simulink model "L4"  (R2016b)
settings: Solver=FixedStepAuto  StartTime=0.0  StopTime=20  FixedStep=0.05  RelTol=1e-3
values from neighbouring files (symbols this model uses):
  global_path_heading = zeros(1,num1)    [referenceline.m]
  global_path_kappa = zeros(1,num1)    [referenceline.m]
  global_path_x = 0: 0.2 : LaneLength    [Map.m]    (also in referenceline.m)
  global_path_y = zeros(1,num1)    [Map.m]    (also in referenceline.m)
(part 1 of 4)
settings Model: Creator=Administrator  LastModifiedBy=Administrator

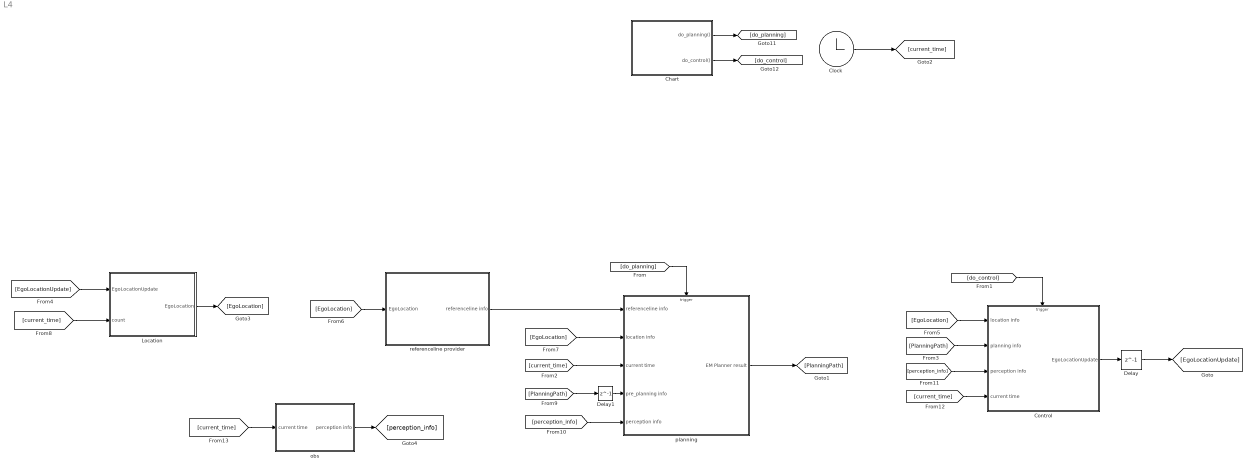
== system L4 ==
  Chart : Stateflow chart  TreatAsAtomicUnit=on
  Clock : Clock
  Control : Subsystem  TreatAsAtomicUnit=on
  Delay : Delay  DelayLength=1  InitialCondition=0
  Delay1 : Delay  DelayLength=1  InitialCondition=0
  Location : Subsystem
  obs : Subsystem
  planning : Subsystem  TreatAsAtomicUnit=on
  referenceline provider : Subsystem
  wires:
  Chart/2(do_control()) -> [do_control]
  Chart/1(do_planning()) -> [do_planning]
  [do_planning] -> planning/Trigger
  [do_control] -> Control/Trigger
  Clock/1 -> [current_time]
  [current_time] -> Location/2(count)
  Control/1(EgoLocationUpdate) -> Delay/1
  [EgoLocationUpdate] -> Location/1(EgoLocationUpdate)
  [PlanningPath] -> Control/2(planning info)
  Location/1(EgoLocation) -> [EgoLocation]
  [EgoLocation] -> Control/1(location info)
  [EgoLocation] -> referenceline provider/1(EgoLocation)
  [EgoLocation] -> planning/2(location info)
  [current_time] -> planning/3(current time)
  referenceline provider/1(referenceline info) -> planning/1(referenceline info)
  planning/1(EM Planner result) -> [PlanningPath]
  [PlanningPath] -> Delay1/1
  Delay1/1 -> planning/4(pre_planning info)
  obs/1(perception info) -> [perception_info]
  [perception_info] -> planning/5(perception info)
  [perception_info] -> Control/3(perception info)
  [current_time] -> Control/4(current time)
  Delay/1 -> [EgoLocationUpdate]
  [current_time] -> obs/1(current time)

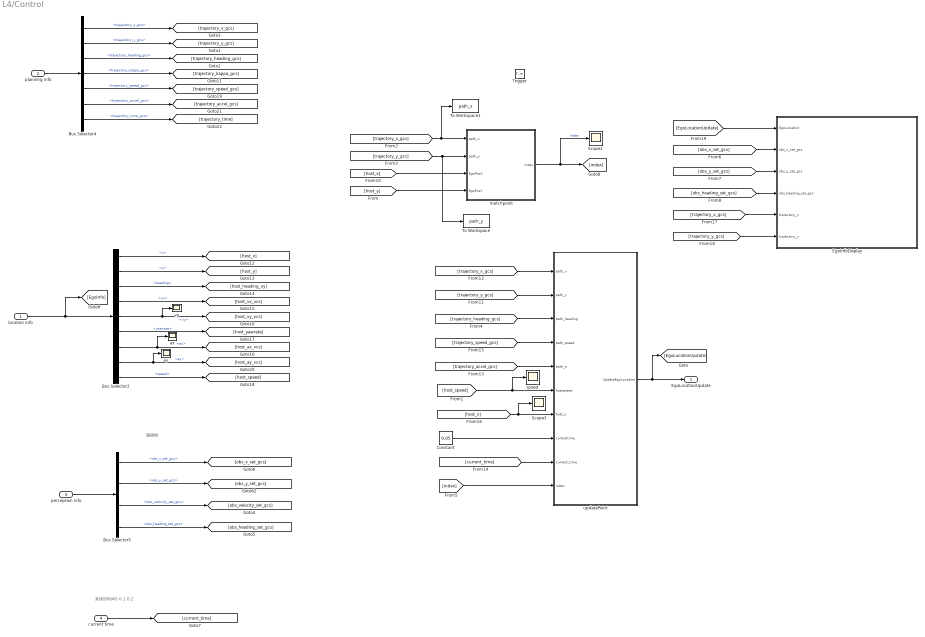
== system L4/Control ==
  note: 障碍物
  note: 系统的时间0 0.1 0.2
  location info : Inport
  planning info : Inport  Port=2
  perception info : Inport  Port=3
  current time : Inport  Port=4
  Trigger : TriggerPort  TriggerType=function-call  VariantControl=Variant
  Bus Selector2 : BusSelector  OutputSignals=x,y,heading,vx,vy,yawrate,ax,ay,speed
  Bus Selector4 : BusSelector  OutputSignals=trajectory_x_gcs,trajectory_y_gcs,trajectory_heading_gcs,trajectory_kappa_gcs,trajectory_speed_gcs,trajectory_accel_gcs,trajectory_time_gcs
  Bus Selector5 : BusSelector  OutputSignals=obs_x_set_gcs,obs_y_set_gcs,obs_velocity_set_gcs,obs_heading_set_gcs
  Constant : Constant  Value=0.05
  EgoInfoDisplay : MATLAB Function  TreatAsAtomicUnit=on
  Scope1 : Scope
  Scope3 : Scope
  To Workspace : ToWorkspace  VariableName=path_y  SampleTime=-1
  To Workspace1 : ToWorkspace  VariableName=path_x  SampleTime=-1
  ax : Scope
  ay : Scope
  matchpoint : MATLAB Function  TreatAsAtomicUnit=on
  speed : Scope
  updatePoint : MATLAB Function  TreatAsAtomicUnit=on
  vy : Scope
  EgoLocationUpdate : Outport
  wires:
  [host_x] -> matchpoint/3(EgoPosX)
  [host_y] -> matchpoint/4(EgoPosY)
  [trajectory_x_gcs] -> To Workspace1/1, matchpoint/1(path_x)
  [trajectory_y_gcs] -> To Workspace/1, matchpoint/2(path_y)
  Constant/1 -> updatePoint/8(controltime)
  [host_speed] -> speed/1, updatePoint/6(hostspeed)
  matchpoint/1(index) -> Scope1/1, [index]  "index"
  [index] -> updatePoint/10(index)
  [trajectory_x_gcs] -> updatePoint/1(path_x)
  [trajectory_y_gcs] -> updatePoint/2(path_y)
  [trajectory_heading_gcs] -> updatePoint/3(path_heading)
  [EgoLocationUpdate] -> EgoInfoDisplay/1(EgoLocation)
  updatePoint/1(UpdateEgoLocation) -> EgoLocationUpdate/1, [EgoLocationUpdate]
  location info/1 -> Bus Selector2/1, [EgoInfo]
  Bus Selector2/2 -> [host_y]  "<y>"
  Bus Selector2/3 -> [host_heading_xy]  "<heading>"
  Bus Selector2/4 -> [host_vx_vcs]  "<vx>"
  Bus Selector2/5 -> vy/1, [host_vy_vcs]  "<vy>"
  Bus Selector2/6 -> [host_yawrate]  "<yawrate>"
  Bus Selector2/7 -> ax/1, [host_ax_vcs]  "<ax>"
  Bus Selector2/8 -> ay/1, [host_ay_vcs]  "<ay>"
  Bus Selector2/1 -> [host_x]  "<x>"
  Bus Selector2/9 -> [host_speed]  "<speed>"
  planning info/1 -> Bus Selector4/1
  Bus Selector4/1 -> [trajectory_x_gcs]  "<trajectory_x_gcs>"
  Bus Selector4/2 -> [trajectory_y_gcs]  "<trajectory_y_gcs>"
  Bus Selector4/3 -> [trajectory_heading_gcs]  "<trajectory_heading_gcs>"
  Bus Selector4/4 -> [trajectory_kappa_gcs]  "<trajectory_kappa_gcs>"
  Bus Selector4/5 -> [trajectory_speed_gcs]  "<trajectory_speed_gcs>"
  Bus Selector4/6 -> [trajectory_accel_gcs]  "<trajectory_accel_gcs>"
  Bus Selector4/7 -> [trajectory_time]  "<trajectory_time_gcs>"
  perception info/1 -> Bus Selector5/1
  Bus Selector5/1 -> [obs_x_set_gcs]  "<obs_x_set_gcs>"
  Bus Selector5/2 -> [obs_y_set_gcs]  "<obs_y_set_gcs>"
  Bus Selector5/3 -> [obs_velocity_set_gcs]  "<obs_velocity_set_gcs>"
  Bus Selector5/4 -> [obs_heading_set_gcs]  "<obs_heading_set_gcs>"
  [obs_x_set_gcs] -> EgoInfoDisplay/2(obs_x_set_gcs)
  [obs_y_set_gcs] -> EgoInfoDisplay/3(obs_y_set_gcs)
  [obs_heading_set_gcs] -> EgoInfoDisplay/4(obs_heading_set_gcs)
  [trajectory_speed_gcs] -> updatePoint/4(path_speed)
  current time/1 -> [current_time]
  [trajectory_accel_gcs] -> updatePoint/5(path_a)
  [host_x] -> Scope3/1, updatePoint/7(host_x)
  [current_time] -> updatePoint/9(current_time)
  [trajectory_x_gcs] -> EgoInfoDisplay/5(trajectory_x)
  [trajectory_y_gcs] -> EgoInfoDisplay/6(trajectory_y)

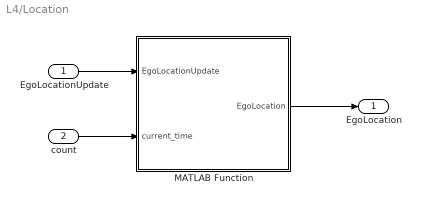
== system L4/Location ==
  EgoLocationUpdate : Inport
  count : Inport  Port=2
  MATLAB Function : MATLAB Function  TreatAsAtomicUnit=on
  EgoLocation : Outport
  wires:
  EgoLocationUpdate/1 -> MATLAB Function/1(EgoLocationUpdate)
  MATLAB Function/1(EgoLocation) -> EgoLocation/1
  count/1 -> MATLAB Function/2(current_time)

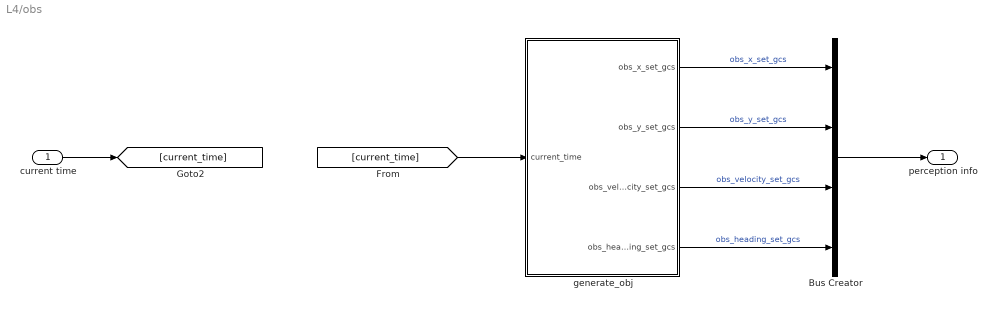
== system L4/obs ==
  current time : Inport
  Bus Creator : BusCreator  Inputs=4
  generate_obj : MATLAB Function  TreatAsAtomicUnit=on
  perception info : Outport
  wires:
  Bus Creator/1 -> perception info/1
  generate_obj/1(obs_x_set_gcs) -> Bus Creator/1  "obs_x_set_gcs"
  generate_obj/2(obs_y_set_gcs) -> Bus Creator/2  "obs_y_set_gcs"
  generate_obj/3(obs_velocity_set_gcs) -> Bus Creator/3  "obs_velocity_set_gcs"
  generate_obj/4(obs_heading_set_gcs) -> Bus Creator/4  "obs_heading_set_gcs"
  current time/1 -> [current_time]
  [current_time] -> generate_obj/1(current_time)

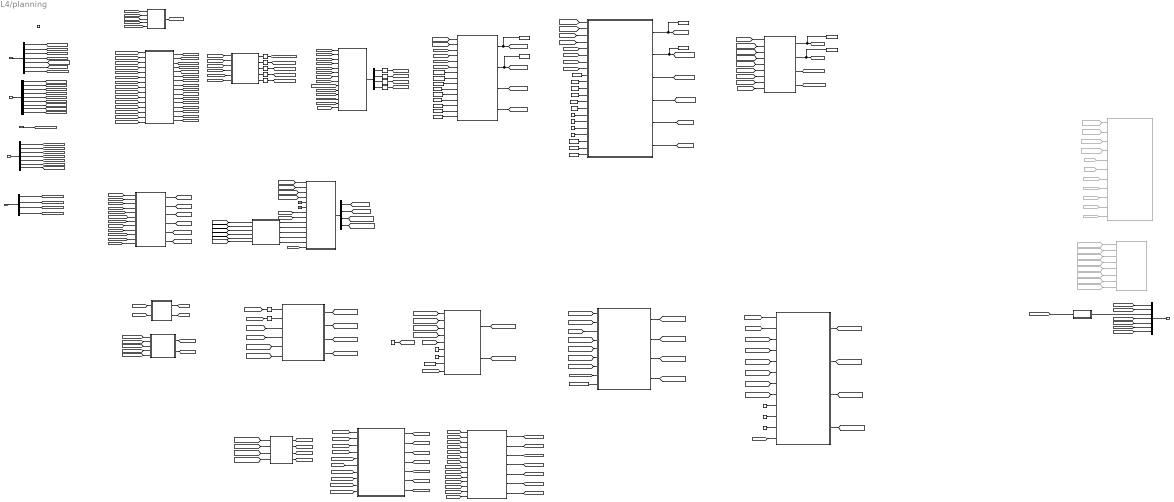
== system L4/planning ==
  note: 障碍物
  note: 规划的起点从世界坐标系转到
      | Frenet坐标系
  note: 世界坐标系下，规划的起点，在referenceline上面
      | 找到最近点。
  note: 函数：获得规划的起点信息，如果控制跟的上就从上一针轨迹的轨迹点
      | step*10+current_time对应的起点。如果控制较差，运动学推理。
      | 此外，拿出来上一个周期之前的轨迹和本次规划的轨迹拼接
  note: 系统的时间0 0.1 0.2
  note: 上一针规划的轨迹
  note: S方向上匹配点值是0
      | 然后后面是负数前面正数
  note: origin_match_point_index是自车在参考线的匹配点
      | origin_x是自车在参考线投影点的坐标x
      | origin_y是自车在参考线投影点的坐标y
  note: 障碍物的处理
      | 静态障碍物SL坐标系
      | 动态障碍物世界坐标系
      | 都是一个点，没有预测轨迹
  note: 动态障碍物的处理
      | 转到SL坐标系
  referenceline info : Inport
  location info : Inport  Port=2
  current time : Inport  Port=3
  pre_planning info : Inport  Port=4
  perception info : Inport  Port=5
  Trigger : TriggerPort  TriggerType=function-call  VariantControl=Variant
  Bus Creator : BusCreator  Inputs=7
  Bus Selector1 : BusSelector  OutputSignals=referenceline_x,referenceline_y,referenceline_heading,referenceline_kappa,origin_match_point_index,origin_x,origin_y
  Bus Selector2 : BusSelector  OutputSignals=x,y,heading,vx,vy,yawrate,ax,ay,speed
  Bus Selector3 : BusSelector  OutputSignals=s_set,l_set,dl_set,ddl_set
  Bus Selector4 : BusSelector  OutputSignals=trajectory_x_gcs,trajectory_y_gcs,trajectory_heading_gcs,trajectory_kappa_gcs,trajectory_speed_gcs,trajectory_accel_gcs,trajectory_time_gcs
  Bus Selector5 : BusSelector  OutputSignals=obs_x_set_gcs,obs_y_set_gcs,obs_velocity_set_gcs,obs_heading_set_gcs
  Bus Selector6 : BusSelector  OutputSignals=s_set,l_set,s_dot_set,l_dot_set
  Cartesian2Frenet : Subsystem
  Cartesian2Frenet1 : Subsystem
  Constant : Constant  Value=1e6
  Constant1 : Constant  Value=1000
  Constant10 : Constant  Value=0.1
  Constant11 : Constant  Value=0.02
  Constant12 : Constant  Value=2
  Constant13 : Constant  Value=25000
  Constant14 : Constant  Value=50
  Constant15 : Constant  Value=20
  Constant16 : Constant  Value=100
  Constant{7,17..19} (4 alike) : Constant  Value=15
  Constant2 : Constant  Value=2
  Constant20 : Constant  Value=3
  Constant21 : Constant  Value=3
  Constant22 : Constant  Value=1.63
  Constant23 : Constant  Value=20
  Constant24 : Constant  Value=4000
  Constant25 : Constant  Value=100
  Constant26 : Constant  Value=10000000
  Constant27 : Constant  Value=0.2*9.8
  Constant28 : Constant  Value=50
  Constant29 : Constant  Value=500
  Constant3 : Constant  Value=3
  Constant4 : Constant  Value=5
  Constant5 : Constant  Value=11
  Constant6 : Constant  Value=4
  Constant8 : Constant  Value=0.5
  Constant9 : Constant  Value=10
  Delay : Delay  DelayLength=1
  Delay1 : Delay  DelayLength=1
  Frenet2Cartesian task : MATLAB Function  TreatAsAtomicUnit=on
  From120 : From  Commented=on  GotoTag=dp_path_s_final
  From124 : From  Commented=on  GotoTag=dp_path_l_final
  From125 : From  Commented=on  GotoTag=l_min
  From126 : From  Commented=on  GotoTag=l_max
  From129 : From  Commented=on  GotoTag=plan_start_l
  From130 : From  Commented=on  GotoTag=plan_start_dl
  From131 : From  Commented=on  GotoTag=plan_start_s
  From132 : From  Commented=on  GotoTag=static_obs_s_set
  From133 : From  Commented=on  GotoTag=static_obs_l_set
  From165 : From  Commented=on  GotoTag=obs_st_s_in_set
  From166 : From  Commented=on  GotoTag=obs_st_s_out_set
  From167 : From  Commented=on  GotoTag=obs_st_t_in_set
  From168 : From  Commented=on  GotoTag=obs_st_t_out_set
  From177 : From  Commented=on  GotoTag=qp_s_init
  From178 : From  Commented=on  GotoTag=relative_time_init
  From71 : From  Commented=on  GotoTag=dp_speed_s
  From73 : From  Commented=on  GotoTag=dp_speed_t
  From91 : From  Commented=on  GotoTag=qp_path_s_final
  From92 : From  Commented=on  GotoTag=qp_path_l_final
  Ground : Ground
  Ground1 : Ground
  MATLAB Function : MATLAB Function  TreatAsAtomicUnit=on
  MATLAB Function1 : MATLAB Function  TreatAsAtomicUnit=on
  MATLAB Function5 : MATLAB Function  Commented=on  TreatAsAtomicUnit=on
  Selector{1..9} (9 alike) : Selector  InputPortWidth=128  IndexOptions=Index vector (dialog)  Indices=1  OutputSizes=1
  To Workspace1 : ToWorkspace  VariableName=qp_trajectory_x  SampleTime=-1
  To Workspace2 : ToWorkspace  VariableName=qp_trajectory_y  SampleTime=-1
  To Workspace3 : ToWorkspace  VariableName=qp_path_s  SampleTime=-1
  To Workspace4 : ToWorkspace  VariableName=qp_path_l  SampleTime=-1
  To Workspace5 : ToWorkspace  VariableName=dp_path_s  SampleTime=-1
  To Workspace6 : ToWorkspace  VariableName=dp_path_l  SampleTime=-1
  calc path length and map between point and s : MATLAB Function  TreatAsAtomicUnit=on
  calc plan start info and stitch trajectory : MATLAB Function  TreatAsAtomicUnit=on
  calc speed planning start condition : MATLAB Function  TreatAsAtomicUnit=on
  dp path decision task : Subsystem
  generate convex space : MATLAB Function  TreatAsAtomicUnit=on
  generate st graph : MATLAB Function  TreatAsAtomicUnit=on
  genrate index to s : MATLAB Function  TreatAsAtomicUnit=on
  increase st point count : MATLAB Function  TreatAsAtomicUnit=on
  match_point : MATLAB Function  TreatAsAtomicUnit=on
  path and speed merge : MATLAB Function  TreatAsAtomicUnit=on
  path planning task : Subsystem
  plot : MATLAB Function  Commented=on  TreatAsAtomicUnit=on
  spee planning with quadratic programming (qp) : MATLAB Function  TreatAsAtomicUnit=on
  speed decision with dynamic planning(dp) : MATLAB Function  TreatAsAtomicUnit=on
  static obs : Subsystem
  stitch trajectory : MATLAB Function  TreatAsAtomicUnit=on
  EM Planner result : Outport
  wires:
  referenceline info/1 -> Bus Selector1/1
  Bus Selector1/1 -> [referenceline_x]  "<referenceline_x>"
  Bus Selector1/2 -> [referenceline_y]  "<referenceline_y>"
  Bus Selector1/3 -> [referenceline_heading]  "<referenceline_heading>"
  Bus Selector1/4 -> [referenceline_kappa]  "<referenceline_kappa>"
  Bus Selector1/5 -> [origin_match_point_index]  "<origin_match_point_index>"
  Bus Selector1/6 -> [origin_x]  "<origin_x>"
  Bus Selector1/7 -> [origin_y]  "<origin_y>"
  [referenceline_x] -> genrate index to s/1(path_x)
  [referenceline_y] -> genrate index to s/2(path_y)
  [origin_x] -> genrate index to s/3(origin_x)
  [origin_y] -> genrate index to s/4(origin_y)
  [origin_match_point_index] -> genrate index to s/5(origin_match_point_index)
  genrate index to s/1(index2s) -> [index2s]
  current time/1 -> [current_time]
  location info/1 -> Bus Selector2/1
  Bus Selector2/2 -> [host_y]  "<y>"
  Bus Selector2/3 -> [host_heading_xy]  "<heading>"
  Bus Selector2/4 -> [host_vx_vcs]  "<vx>"
  Bus Selector2/5 -> [host_vy_vcs]  "<vy>"
  Bus Selector2/6 -> [host_yawrate]  "<yawrate>"
  Bus Selector2/7 -> [host_ax_vcs]  "<ax>"
  Bus Selector2/8 -> [host_ay_vcs]  "<ay>"
  Bus Selector2/1 -> [host_x]  "<x>"
  Bus Selector2/9 -> [host_speed]  "<speed>"
  [host_ay_vcs] -> calc plan start info and stitch trajectory/15(host_ay)
  [host_ax_vcs] -> calc plan start info and stitch trajectory/14(host_ax)
  [host_vy_vcs] -> calc plan start info and stitch trajectory/13(host_vy)
  [host_vx_vcs] -> calc plan start info and stitch trajectory/12(host_vx)
  [host_heading_xy] -> calc plan start info and stitch trajectory/11(host_heading_xy)
  [host_y] -> calc plan start info and stitch trajectory/10(host_y)
  [host_x] -> calc plan start info and stitch trajectory/9(host_x)
  [current_time] -> calc plan start info and stitch trajectory/8(current_time)
  [pre_trajectory_x_gcs] -> calc plan start info and stitch trajectory/1(pre_trajectory_x)
  [pre_trajectory_y_gcs] -> calc plan start info and stitch trajectory/2(pre_trajectory_y)
  [pre_trajectory_time] -> calc plan start info and stitch trajectory/7(pre_trajectory_time)
  [pre_trajectory_accel_gcs] -> calc plan start info and stitch trajectory/6(pre_trajectory_accel)
  [pre_trajectory_speed_gcs] -> calc plan start info and stitch trajectory/5(pre_trajectory_velocity)
  [pre_trajectory_kappa_gcs] -> calc plan start info and stitch trajectory/4(pre_trajectory_kappa)
  [pre_trajectory_heading_gcs] -> calc plan start info and stitch trajectory/3(pre_trajectory_heading)
  calc plan start info and stitch trajectory/1(plan_start_x) -> [plan_start_x_gcs]
  calc plan start info and stitch trajectory/2(plan_start_y) -> [plan_start_y_gcs]
  calc plan start info and stitch trajectory/3(plan_start_heading) -> [plan_start_heading_gcs]
  calc plan start info and stitch trajectory/4(plan_start_kappa) -> [plan_start_kappa_gcs]
  calc plan start info and stitch trajectory/5(plan_start_vx) -> [plan_start_vx_gcs]
  calc plan start info and stitch trajectory/6(plan_start_vy) -> [plan_start_vy_gcs]
  calc plan start info and stitch trajectory/7(plan_start_ax) -> [plan_start_ax_gcs]
  calc plan start info and stitch trajectory/8(plan_start_ay) -> [plan_start_ay_gcs]
  calc plan start info and stitch trajectory/9(plan_start_time) -> [plan_start_time]
  calc plan start info and stitch trajectory/10(stitch_x) -> [stitch_x_gcs]
  calc plan start info and stitch trajectory/11(stitch_y) -> [stitch_y_gcs]
  calc plan start info and stitch trajectory/12(stitch_heading) -> [stitch_heading_gcs]
  calc plan start info and stitch trajectory/13(stitch_kappa) -> [stitch_kappa_gcs]
  calc plan start info and stitch trajectory/14(stitch_speed) -> [stitch_speed_gcs]
  calc plan start info and stitch trajectory/15(stitch_accel) -> [stitch_accel_gcs]
  calc plan start info and stitch trajectory/16(stitch_time) -> [stitch_time]
  pre_planning info/1 -> Bus Selector4/1
  Bus Selector4/1 -> [pre_trajectory_x_gcs]  "<trajectory_x_gcs>"
  Bus Selector4/2 -> [pre_trajectory_y_gcs]  "<trajectory_y_gcs>"
  Bus Selector4/3 -> [pre_trajectory_heading_gcs]  "<trajectory_heading_gcs>"
  Bus Selector4/4 -> [pre_trajectory_kappa_gcs]  "<trajectory_kappa_gcs>"
  Bus Selector4/5 -> [pre_trajectory_speed_gcs]  "<trajectory_speed_gcs>"
  Bus Selector4/6 -> [pre_trajectory_accel_gcs]  "<trajectory_accel_gcs>"
  Bus Selector4/7 -> [pre_trajectory_time]  "<trajectory_time_gcs>"
  match_point/5(proj_kappa_set) -> Selector5/1
  match_point/3(proj_y_set) -> Selector3/1
  match_point/1(match_point_index_set) -> Selector1/1
  match_point/4(proj_heading_set) -> Selector4/1
  match_point/2(proj_x_set) -> Selector2/1
  [plan_start_x_gcs] -> match_point/1(x_set)
  [plan_start_y_gcs] -> match_point/2(y_set)
  [referenceline_x] -> match_point/3(frenet_path_x)
  [referenceline_y] -> match_point/4(frenet_path_y)
  [referenceline_heading] -> match_point/5(frenet_path_heading)
  [referenceline_kappa] -> match_point/6(frenet_path_kappa)
  Selector1/1 -> [plan_start_match_point_index]
  Selector2/1 -> [plan_start_proj_x]
  Selector3/1 -> [plan_start_proj_y]
  Selector4/1 -> [plan_start_proj_heading]
  Selector5/1 -> [plan_start_proj_kappa]
  [plan_start_y_gcs] -> Cartesian2Frenet/2(y_set)
  [plan_start_x_gcs] -> Cartesian2Frenet/1(x_set)
  [plan_start_vx_gcs] -> Cartesian2Frenet/3(vx_set)
  [plan_start_vy_gcs] -> Cartesian2Frenet/4(vy_set)
  [plan_start_ax_gcs] -> Cartesian2Frenet/5(ax_set)
  [plan_start_ay_gcs] -> Cartesian2Frenet/6(ay_set)
  [referenceline_x] -> Cartesian2Frenet/7(frenet_path_x)
  [referenceline_y] -> Cartesian2Frenet/8(frenet_path_y)
  [plan_start_match_point_index] -> Cartesian2Frenet/9(proj_match_point_index_set)
  [plan_start_proj_x] -> Cartesian2Frenet/10(proj_x_set)
  [plan_start_proj_y] -> Cartesian2Frenet/11(proj_y_set)
  [plan_start_proj_heading] -> Cartesian2Frenet/12(proj_heading_set)
  [plan_start_proj_kappa] -> Cartesian2Frenet/13(proj_kappa_set)
  Cartesian2Frenet/1(Cartesian2FrenetOut) -> Bus Selector3/1
  Bus Selector3/4 -> Selector9/1  "<ddl_set>"
  Bus Selector3/3 -> Selector8/1  "<dl_set>"
  Bus Selector3/2 -> Selector7/1  "<l_set>"
  Bus Selector3/1 -> Selector6/1  "<s_set>"
  Selector6/1 -> [plan_start_s]
  Selector7/1 -> [plan_start_l]
  Selector8/1 -> [plan_start_dl]
  Selector9/1 -> [plan_start_ddl]
  [index2s] -> Cartesian2Frenet/14(index2s)
  dp path decision task/2(dp_path_l_final) -> To Workspace6/1, [dp_path_l_final]
  dp path decision task/3(dp_path_dl_final) -> [dp_path_dl_final]
  dp path decision task/4(dp_path_ddl_final) -> [dp_path_ddl_final]
  [static_obs_s_set] -> dp path decision task/1(static_obs_s_set)
  [static_obs_l_set] -> dp path decision task/2(static_obs_l_set)
  [plan_start_ddl] -> dp path decision task/6(plan_start_ddl)
  [plan_start_dl] -> dp path decision task/5(plan_start_dl)
  [plan_start_l] -> dp path decision task/4(plan_start_l)
  [plan_start_s] -> dp path decision task/3(plan_start_s)
  Constant8/1 -> dp path decision task/15(dp_sample_l)
  Constant7/1 -> dp path decision task/14(dp_sample_s)
  Constant6/1 -> dp path decision task/13(dp_col)
  Constant5/1 -> dp path decision task/12(dp_row)
  Constant4/1 -> dp path decision task/11(dp_cost_ref)
  Constant3/1 -> dp path decision task/10(dp_cost_dddl)
  Constant/1 -> dp path decision task/7(dp_cost_collision)
  Constant1/1 -> dp path decision task/8(dp_cost_dl)
  Constant2/1 -> dp path decision task/9(dp_cost_ddl)
  [host_x] -> static obs/1(host_x)
  [host_y] -> static obs/2(host_y)
  [host_heading_xy] -> static obs/3(host_heading_xy)
  [obs_x_set_gcs] -> static obs/4(obs_x_set_gcs)
  [obs_y_set_gcs] -> static obs/5(obs_y_set_gcs)
  [obs_velocity_set_gcs] -> static obs/6(obs_velocity_set_gcs)
  [obs_heading_set_gcs] -> static obs/7(obs_heading_set_gcs)
  [referenceline_x] -> static obs/8(referenceline_x)
  [referenceline_y] -> static obs/9(referenceline_y)
  [referenceline_heading] -> static obs/10(referenceline_heading)
  [referenceline_kappa] -> static obs/11(referenceline_kappa)
  [index2s] -> static obs/12(index2s)
  static obs/1(static_obs_s_set) -> [static_obs_s_set]
  static obs/2(static_obs_l_set) -> [static_obs_l_set]
  static obs/3(dynamic_obs_x_set) -> [dynamic_obs_x_set]
  static obs/4(dynamic_obs_y_set) -> [dynamic_obs_y_set]
  static obs/5(dynamic_obs_vx_set) -> [dynamic_obs_vx_set]
  static obs/6(dynamic_obs_vy_set) -> [dynamic_obs_vy_set]
  perception info/1 -> Bus Selector5/1
  Bus Selector5/1 -> [obs_x_set_gcs]  "<obs_x_set_gcs>"
  Bus Selector5/2 -> [obs_y_set_gcs]  "<obs_y_set_gcs>"
  Bus Selector5/3 -> [obs_velocity_set_gcs]  "<obs_velocity_set_gcs>"
  Bus Selector5/4 -> [obs_heading_set_gcs]  "<obs_heading_set_gcs>"
  [dynamic_obs_vy_set] -> Cartesian2Frenet1/4(vy_set)
  [dynamic_obs_vx_set] -> Cartesian2Frenet1/3(vx_set)
  [dynamic_obs_y_set] -> Cartesian2Frenet1/2(y_set)
  [dynamic_obs_x_set] -> Cartesian2Frenet1/1(x_set)
  Ground/1 -> Cartesian2Frenet1/5(ax_set)
  Ground1/1 -> Cartesian2Frenet1/6(ay_set)
  [trajectory_x_init] -> Cartesian2Frenet1/7(frenet_path_x)
  [trajectory_y_init] -> Cartesian2Frenet1/8(frenet_path_y)
  MATLAB Function1/1(match_point_index_set) -> Cartesian2Frenet1/9(proj_match_point_index_set)
  MATLAB Function1/2(proj_x_set) -> Cartesian2Frenet1/10(proj_x_set)
  MATLAB Function1/3(proj_y_set) -> Cartesian2Frenet1/11(proj_y_set)
  MATLAB Function1/4(proj_heading_set) -> Cartesian2Frenet1/12(proj_heading_set)
  MATLAB Function1/5(proj_kappa_set) -> Cartesian2Frenet1/13(proj_kappa_set)
  [trajectory_x_init] -> MATLAB Function1/3(frenet_path_x)
  [trajectory_y_init] -> MATLAB Function1/4(frenet_path_y)
  [trajectory_heading_init] -> MATLAB Function1/5(frenet_path_heading)
  [trajectory_kappa_init] -> MATLAB Function1/6(frenet_path_kappa)
  [dynamic_obs_y_set] -> MATLAB Function1/2(y_set)
  [dynamic_obs_x_set] -> MATLAB Function1/1(x_set)
  Cartesian2Frenet1/1(Cartesian2FrenetOut) -> Bus Selector6/1
  Bus Selector6/1 -> [dynamic_obs_s_set]  "<s_set>"
  Bus Selector6/2 -> [dynamic_obs_l_set]  "<l_set>"
  Bus Selector6/3 -> [dynamic_obs_s_dot_set]  "<s_dot_set>"
  Bus Selector6/4 -> [dynamic_obs_l_dot_set]  "<l_dot_set>"
  [path_index2s] -> Cartesian2Frenet1/14(index2s)
  [index2s] -> Frenet2Cartesian task/9(index2s)
  [referenceline_x] -> Frenet2Cartesian task/5(frenet_path_x)
  [referenceline_y] -> Frenet2Cartesian task/6(frenet_path_y)
  [referenceline_heading] -> Frenet2Cartesian task/7(frenet_path_heading)
  [referenceline_kappa] -> Frenet2Cartesian task/8(frenet_path_kappa)
  Frenet2Cartesian task/1(x_set) -> To Workspace1/1, [trajectory_x_init]
  Frenet2Cartesian task/2(y_set) -> To Workspace2/1, [trajectory_y_init]
  Frenet2Cartesian task/3(heading_set) -> [trajectory_heading_init]
  Frenet2Cartesian task/4(kappa_set) -> [trajectory_kappa_init]
  [qp_path_ddl_final] -> Frenet2Cartesian task/4(ddl_set)
  [qp_path_l_final] -> Frenet2Cartesian task/2(l_set)
  [qp_path_dl_final] -> Frenet2Cartesian task/3(dl_set)
  [qp_path_s_final] -> Frenet2Cartesian task/1(s_set)
  [dp_path_s_final] -> path planning task/1(dp_path_s_final)
  [dp_path_l_final] -> path planning task/2(dp_path_l_final)
  [plan_start_l] -> path planning task/6(plan_start_l)
  [plan_start_ddl] -> path planning task/8(plan_start_ddl)
  [plan_start_dl] -> path planning task/7(plan_start_dl)
  Constant22/1 -> path planning task/19(host_w)
  Constant21/1 -> path planning task/18(host_d2)
  Constant20/1 -> path planning task/17(host_d1)
  Constant19/1 -> path planning task/16(qp_cost_end_ddl)
  Constant18/1 -> path planning task/15(qp_cost_end_dl)
  Constant17/1 -> path planning task/14(qp_cost_endl)
  Constant16/1 -> path planning task/13(qp_cost_centre)
  Constant15/1 -> path planning task/12(qp_cost_dddl)
  Constant14/1 -> path planning task/11(qp_cost_ddl)
  Constant13/1 -> path planning task/10(qp_cost_dl)
  Constant12/1 -> path planning task/9(qp_cost_l)
  [static_obs_s_set] -> path planning task/3(static_obs_s_set)
  [static_obs_l_set] -> path planning task/4(static_obs_l_set)
  Constant10/1 -> path planning task/20(delta_dl_max)
  Constant11/1 -> path planning task/21(delta_ddl_max)
  path planning task/1(qp_path_s_final) -> To Workspace3/1, [qp_path_s_final]
  path planning task/2(qp_path_l_final) -> To Workspace4/1, [qp_path_l_final]
  path planning task/3(qp_path_dl_final) -> [qp_path_dl_final]
  path planning task/4(qp_path_ddl_final) -> [qp_path_ddl_final]
  [plan_start_s] -> path planning task/5(plan_start_s)
  calc path length and map between point and s/2(path_index2s) -> [path_index2s]
  calc path length and map between point and s/1(path_s_end) -> [path_s_end]
  [trajectory_y_init] -> calc path length and map between point and s/2(trajectory_y)
  [trajectory_x_init] -> calc path length and map between point and s/1(trajectory_x)
  [plan_start_vy_gcs] -> calc speed planning start condition/2(plan_start_vy)
  [plan_start_heading_gcs] -> calc speed planning start condition/5(plan_start_heading)
  [plan_start_ax_gcs] -> calc speed planning start condition/3(plan_start_ax)
  calc speed planning start condition/1(plan_start_s_dot) -> [plan_start_s_dot]
  [plan_start_ay_gcs] -> calc speed planning start condition/4(plan_start_ay)
  [plan_start_vx_gcs] -> calc speed planning start condition/1(plan_start_vx)
  calc speed planning start condition/2(plan_start_s_dot2) -> [plan_start_s_dot2]
  [s] -> Delay/1
  [relative_time] -> Delay1/1
  Delay/1 -> generate st graph/1(pre_trajectory_s)
  Delay1/1 -> generate st graph/2(pre_trajectory_t)
  [dynamic_obs_s_set] -> generate st graph/3(dynamic_obs_s_set)
  [dynamic_obs_l_set] -> generate st graph/4(dynamic_obs_l_set)
  [dynamic_obs_s_dot_set] -> generate st graph/5(dynamic_obs_s_dot_set)
  [dynamic_obs_l_dot_set] -> generate st graph/6(dynamic_obs_l_dot_set)
  generate st graph/1(obs_st_s_in_set) -> [obs_st_s_in_set]
  generate st graph/3(obs_st_t_in_set) -> [obs_st_t_in_set]
  generate st graph/4(obs_st_t_out_set) -> [obs_st_t_out_set]
  generate st graph/2(obs_st_s_out_set) -> [obs_st_s_out_set]
  [obs_st_s_in_set] -> speed decision with dynamic planning(dp)/1(obs_st_s_in_set)
  [obs_st_s_out_set] -> speed decision with dynamic planning(dp)/2(obs_st_s_out_set)
  [obs_st_t_in_set] -> speed decision with dynamic planning(dp)/3(obs_st_t_in_set)
  [obs_st_t_out_set] -> speed decision with dynamic planning(dp)/4(obs_st_t_out_set)
  Constant24/1 -> speed decision with dynamic planning(dp)/6(w_cost_ref_speed)
  Constant25/1 -> speed decision with dynamic planning(dp)/7(w_cost_accel)
  Constant26/1 -> speed decision with dynamic planning(dp)/8(w_cost_obs)
  [plan_start_s_dot] -> speed decision with dynamic planning(dp)/9(plan_start_s_dot)
  speed decision with dynamic planning(dp)/2(dp_speed_t) -> [dp_speed_t]
  speed decision with dynamic planning(dp)/1(dp_speed_s) -> [dp_speed_s]
  Constant23/1 -> [reference_speed]
  [reference_speed] -> speed decision with dynamic planning(dp)/5(reference_speed_unlimit)
  [path_index2s] -> generate convex space/3(path_index2s)
  [dp_speed_s] -> generate convex space/1(dp_speed_s)
  [dp_speed_t] -> generate convex space/2(dp_speed_t)
  [obs_st_s_in_set] -> generate convex space/4(obs_st_s_in_set)
  [obs_st_t_out_set] -> generate convex space/7(obs_st_t_out_set)
  [obs_st_t_in_set] -> generate convex space/6(obs_st_t_in_set)
  [obs_st_s_out_set] -> generate convex space/5(obs_st_s_out_set)
  [trajectory_kappa_init] -> generate convex space/8(trajectory_kappa_init)
  Constant27/1 -> generate convex space/9(max_lateral_accel)
  generate convex space/1(s_lb) -> [s_lb]
  generate convex space/2(s_ub) -> [s_ub]
  generate convex space/3(s_dot_lb) -> [s_dot_lb]
  generate convex space/4(s_dot_ub) -> [s_dot_ub]
  [plan_start_s_dot] -> spee planning with quadratic programming (qp)/1(plan_start_s_dot)
  [dp_speed_s] -> spee planning with quadratic programming (qp)/3(dp_speed_s)
  [dp_speed_t] -> spee planning with quadratic programming (qp)/4(dp_speed_t)
  [s_lb] -> spee planning with quadratic programming (qp)/5(s_lb)
  [s_ub] -> spee planning with quadratic programming (qp)/6(s_ub)
  [s_dot_lb] -> spee planning with quadratic programming (qp)/7(s_dot_lb)
  [s_dot_ub] -> spee planning with quadratic programming (qp)/8(s_dot_ub)
  spee planning with quadratic programming (qp)/1(qp_s_init) -> [qp_s_init]
  spee planning with quadratic programming (qp)/2(qp_s_dot_init) -> [qp_s_dot_init]
  spee planning with quadratic programming (qp)/3(qp_s_dot2_init) -> [qp_s_dot2_init]
  spee planning with quadratic programming (qp)/4(relative_time_init) -> [relative_time_init]
  Constant9/1 -> spee planning with quadratic programming (qp)/9(w_cost_s_dot2)
  Constant28/1 -> spee planning with quadratic programming (qp)/10(w_cost_v_ref)
  Constant29/1 -> spee planning with quadratic programming (qp)/11(w_cost_jerk)
  [plan_start_s_dot2] -> spee planning with quadratic programming (qp)/2(plan_start_s_dot2)
  [reference_speed] -> spee planning with quadratic programming (qp)/12(speed_reference)
  path and speed merge/7(trajectory_time) -> [trajectory_time]
  path and speed merge/1(trajectory_x) -> [trajectory_x]
  [trajectory_speed] -> stitch trajectory/5(trajectory_speed)
  path and speed merge/4(trajectory_kappa) -> [trajectory_kappa]
  [stitch_time] -> stitch trajectory/14(stitch_time)
  stitch trajectory/4(trajectory_kappa_final) -> [trajectory_kappa_final]
  [stitch_speed_gcs] -> stitch trajectory/12(stitch_speed)
  [stitch_x_gcs] -> stitch trajectory/8(stitch_x)
  stitch trajectory/1(trajectory_x_final) -> [trajectory_x_final]
  [stitch_heading_gcs] -> stitch trajectory/10(stitch_heading)
  [stitch_y_gcs] -> stitch trajectory/9(stitch_y)
  stitch trajectory/6(trajectory_accel_final) -> [trajectory_accel_final]
  [trajectory_accel] -> stitch trajectory/6(trajectory_accel)
  [trajectory_kappa] -> stitch trajectory/4(trajectory_kappa)
  [trajectory_x_init] -> path and speed merge/7(trajectory_x_init)
  stitch trajectory/2(trajectory_y_final) -> [trajectory_y_final]
  stitch trajectory/3(trajectory_heading_final) -> [trajectory_heading_final]
  path and speed merge/3(trajectory_heading) -> [trajectory_heading]
  stitch trajectory/5(trajectory_speed_final) -> [trajectory_speed_final]
  [trajectory_y] -> stitch trajectory/2(trajectory_y)
  [trajectory_kappa_init] -> path and speed merge/10(trajectory_kappa_init)
  [stitch_accel_gcs] -> stitch trajectory/13(stitch_accel)
  [trajectory_x] -> stitch trajectory/1(trajectory_x)
  path and speed merge/6(trajectory_accel) -> [trajectory_accel]
  [stitch_kappa_gcs] -> stitch trajectory/11(stitch_kappa)
  [path_index2s] -> path and speed merge/6(path_s)
  path and speed merge/2(trajectory_y) -> [trajectory_y]
  [trajectory_heading_init] -> path and speed merge/9(trajectory_heading_init)
  [plan_start_time] -> path and speed merge/5(current_time)
  path and speed merge/5(trajectory_speed) -> [trajectory_speed]
  [trajectory_y_init] -> path and speed merge/8(trajectory_y_init)
  [trajectory_time] -> stitch trajectory/7(trajectory_time)
  [trajectory_heading] -> stitch trajectory/3(trajectory_heading)
  increase st point count/3(s_dot2) -> [s_dot2]
  increase st point count/2(s_dot) -> [s_dot]
  increase st point count/1(s) -> [s]
  increase st point count/4(relative_time) -> [relative_time]
  [s_dot] -> path and speed merge/2(s_dot)
  [s] -> path and speed merge/1(s)
  [s_dot2] -> path and speed merge/3(s_dot2)
  [relative_time] -> path and speed merge/4(relative_time)
  stitch trajectory/7(trajectory_time_final) -> [trajectory_time_final]
  [qp_s_init] -> increase st point count/1(s_init)
  [qp_s_dot2_init] -> increase st point count/3(s_dot2_init)
  [qp_s_dot_init] -> increase st point count/2(s_dot_init)
  [relative_time_init] -> increase st point count/4(relative_time_init)
  Bus Creator/1 -> EM Planner result/1
  [trajectory_x_final] -> Bus Creator/1  "trajectory_x_gcs"
  [trajectory_time_final] -> Bus Creator/7  "trajectory_time_gcs"
  [trajectory_accel_final] -> Bus Creator/6  "trajectory_accel_gcs"
  [trajectory_speed_final] -> Bus Creator/5  "trajectory_speed_gcs"
  [trajectory_heading_final] -> MATLAB Function/1(trajectory_heading_final)
  [trajectory_kappa_final] -> Bus Creator/4  "trajectory_kappa_gcs"
  [trajectory_y_final] -> Bus Creator/2  "trajectory_y_gcs"
  From120/1 -> plot/1(dp_s)
  From124/1 -> plot/2(dp_l)
  From125/1 -> plot/5(l_min)
  From126/1 -> plot/6(l_max)
  From130/1 -> plot/11(start_dl)
  From129/1 -> plot/10(start_l)
  From131/1 -> plot/9(start_s)
  From132/1 -> plot/7(obs_s_set)
  From133/1 -> plot/8(obs_l_set)
  From91/1 -> plot/3(qp_s)
  From92/1 -> plot/4(qp_l)
  MATLAB Function/1(y) -> Bus Creator/3  "trajectory_heading_gcs"
  From165/1 -> MATLAB Function5/5(obs_s_in_set)
  From166/1 -> MATLAB Function5/6(obs_s_out_set)
  From167/1 -> MATLAB Function5/7(obs_t_in_set)
  From168/1 -> MATLAB Function5/8(obs_t_out_set)
  From73/1 -> MATLAB Function5/2(dp_speed_t)
  From71/1 -> MATLAB Function5/1(dp_speed_s)
  From177/1 -> MATLAB Function5/3(qp_speed_s)
  From178/1 -> MATLAB Function5/4(qp_speed_t)
  path planning task/5(Lmin) -> [l_min]
  path planning task/6(Lmax) -> [l_max]
  dp path decision task/1(dp_path_s_final) -> To Workspace5/1, [dp_path_s_final]

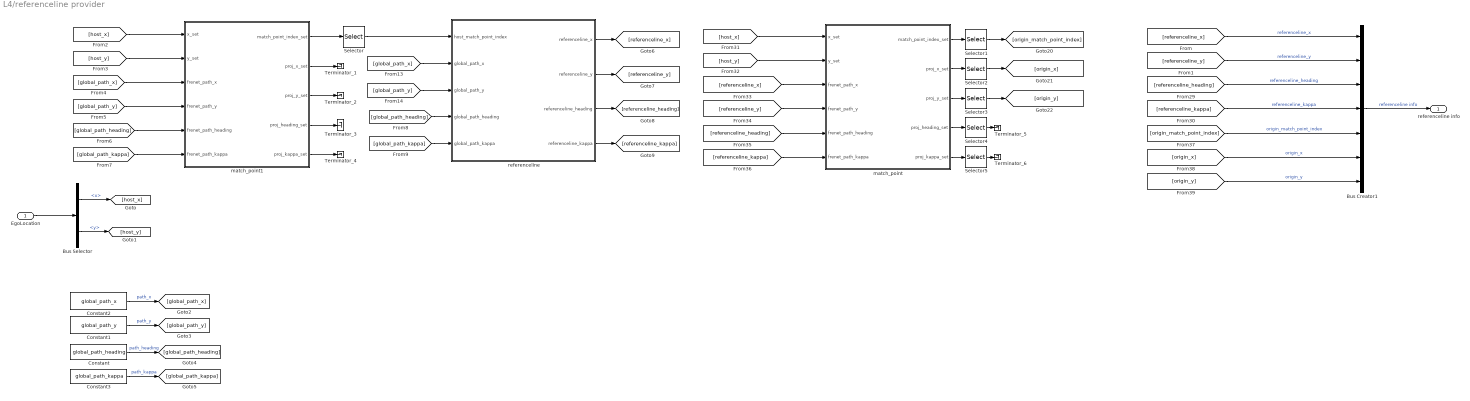
== system L4/referenceline provider ==
  EgoLocation : Inport
  Bus Creator1 : BusCreator  Inputs=7
  Bus Selector : BusSelector  OutputSignals=x,y
  Constant : Constant  Value=global_path_heading
  Constant1 : Constant  Value=global_path_y
  Constant2 : Constant  Value=global_path_x
  Constant3 : Constant  Value=global_path_kappa
  Selector{,1..5} (6 alike) : Selector  InputPortWidth=128  IndexOptions=Index vector (dialog)  Indices=1  OutputSizes=1
  Terminator_{1..6} (6 alike) : Terminator
  match_point : MATLAB Function  TreatAsAtomicUnit=on
  match_point1 : MATLAB Function  TreatAsAtomicUnit=on
  referenceline : MATLAB Function  TreatAsAtomicUnit=on
  referenceline info : Outport
  wires:
  [host_x] -> match_point/1(x_set)
  [host_y] -> match_point/2(y_set)
  [referenceline_x] -> match_point/3(frenet_path_x)
  [referenceline_y] -> match_point/4(frenet_path_y)
  [referenceline_heading] -> match_point/5(frenet_path_heading)
  [referenceline_kappa] -> match_point/6(frenet_path_kappa)
  match_point/1(match_point_index_set) -> Selector1/1
  match_point/2(proj_x_set) -> Selector2/1
  match_point/3(proj_y_set) -> Selector3/1
  match_point/4(proj_heading_set) -> Selector4/1
  match_point/5(proj_kappa_set) -> Selector5/1
  Selector1/1 -> [origin_match_point_index]
  Selector2/1 -> [origin_x]
  Selector3/1 -> [origin_y]
  Selector4/1 -> Terminator_5/1
  Selector5/1 -> Terminator_6/1
  [referenceline_x] -> Bus Creator1/1  "referenceline_x"
  [referenceline_y] -> Bus Creator1/2  "referenceline_y"
  Bus Creator1/1 -> referenceline info/1  "referenceline info"
  [referenceline_kappa] -> Bus Creator1/4  "referenceline_kappa"
  [referenceline_heading] -> Bus Creator1/3  "referenceline_heading"
  [origin_match_point_index] -> Bus Creator1/5  "origin_match_point_index"
  [origin_x] -> Bus Creator1/6  "origin_x"
  [origin_y] -> Bus Creator1/7  "origin_y"
  EgoLocation/1 -> Bus Selector/1
  Bus Selector/1 -> [host_x]  "<x>"
  Bus Selector/2 -> [host_y]  "<y>"
  [host_y] -> match_point1/2(y_set)
  [host_x] -> match_point1/1(x_set)
  match_point1/2(proj_x_set) -> Terminator_1/1
  match_point1/3(proj_y_set) -> Terminator_2/1
  match_point1/4(proj_heading_set) -> Terminator_3/1
  match_point1/5(proj_kappa_set) -> Terminator_4/1
  [global_path_x] -> referenceline/2(global_path_x)
  Selector/1 -> referenceline/1(host_match_point_index)
  [global_path_y] -> referenceline/3(global_path_y)
  match_point1/1(match_point_index_set) -> Selector/1
  Constant2/1 -> [global_path_x]  "path_x"
  Constant1/1 -> [global_path_y]  "path_y"
  [global_path_y] -> match_point1/4(frenet_path_y)
  [global_path_x] -> match_point1/3(frenet_path_x)
  Constant/1 -> [global_path_heading]  "path_heading"
  Constant3/1 -> [global_path_kappa]  "path_kappa"
  [global_path_heading] -> match_point1/5(frenet_path_heading)
  [global_path_kappa] -> match_point1/6(frenet_path_kappa)
  [global_path_heading] -> referenceline/4(global_path_heading)
  [global_path_kappa] -> referenceline/5(global_path_kappa)
  referenceline/1(referenceline_x) -> [referenceline_x]
  referenceline/4(referenceline_kappa) -> [referenceline_kappa]
  referenceline/3(referenceline_heading) -> [referenceline_heading]
  referenceline/2(referenceline_y) -> [referenceline_y]

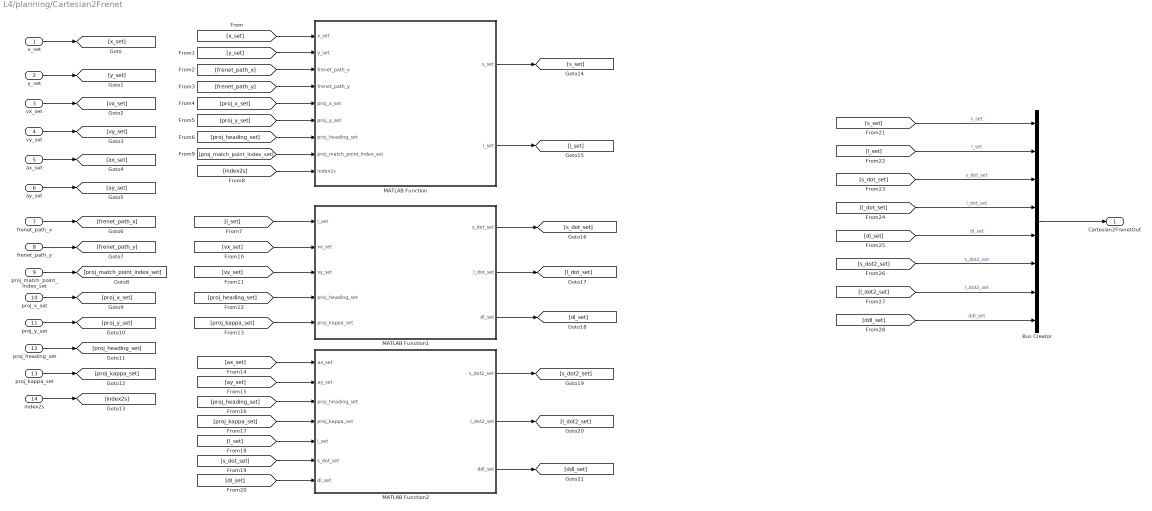
== system L4/planning/Cartesian2Frenet ==
  x_set : Inport
  y_set : Inport  Port=2
  vx_set : Inport  Port=3
  vy_set : Inport  Port=4
  ax_set : Inport  Port=5
  ay_set : Inport  Port=6
  frenet_path_x : Inport  Port=7
  frenet_path_y : Inport  Port=8
  proj_match_point_index_set : Inport  Port=9
  proj_x_set : Inport  Port=10
  proj_y_set : Inport  Port=11
  proj_heading_set : Inport  Port=12
  proj_kappa_set : Inport  Port=13
  index2s : Inport  Port=14
  Bus Creator : BusCreator  Inputs=8
  MATLAB Function : MATLAB Function  TreatAsAtomicUnit=on
  MATLAB Function1 : MATLAB Function  TreatAsAtomicUnit=on
  MATLAB Function2 : MATLAB Function  TreatAsAtomicUnit=on
  Cartesian2FrenetOut : Outport
  wires:
  x_set/1 -> [x_set]
  y_set/1 -> [y_set]
  vx_set/1 -> [vx_set]
  vy_set/1 -> [vy_set]
  ax_set/1 -> [ax_set]
  ay_set/1 -> [ay_set]
  frenet_path_x/1 -> [frenet_path_x]
  frenet_path_y/1 -> [frenet_path_y]
  proj_match_point_index_set/1 -> [proj_match_point_index_set]
  proj_x_set/1 -> [proj_x_set]
  proj_y_set/1 -> [proj_y_set]
  proj_heading_set/1 -> [proj_heading_set]
  proj_kappa_set/1 -> [proj_kappa_set]
  index2s/1 -> [index2s]
  [x_set] -> MATLAB Function/1(x_set)
  [y_set] -> MATLAB Function/2(y_set)
  [frenet_path_x] -> MATLAB Function/3(frenet_path_x)
  [frenet_path_y] -> MATLAB Function/4(frenet_path_y)
  [proj_x_set] -> MATLAB Function/5(proj_x_set)
  [proj_match_point_index_set] -> MATLAB Function/8(proj_match_point_index_set)
  [proj_y_set] -> MATLAB Function/6(proj_y_set)
  [proj_heading_set] -> MATLAB Function/7(proj_heading_set)
  [index2s] -> MATLAB Function/9(index2s)
  MATLAB Function/1(s_set) -> [s_set]
  MATLAB Function/2(l_set) -> [l_set]
  [l_set] -> MATLAB Function1/1(l_set)
  [vx_set] -> MATLAB Function1/2(vx_set)
  [vy_set] -> MATLAB Function1/3(vy_set)
  [proj_heading_set] -> MATLAB Function1/4(proj_heading_set)
  [proj_kappa_set] -> MATLAB Function1/5(proj_kappa_set)
  [ax_set] -> MATLAB Function2/1(ax_set)
  [ay_set] -> MATLAB Function2/2(ay_set)
  [proj_heading_set] -> MATLAB Function2/3(proj_heading_set)
  [proj_kappa_set] -> MATLAB Function2/4(proj_kappa_set)
  [l_set] -> MATLAB Function2/5(l_set)
  MATLAB Function1/1(s_dot_set) -> [s_dot_set]
  MATLAB Function1/2(l_dot_set) -> [l_dot_set]
  MATLAB Function1/3(dl_set) -> [dl_set]
  [s_dot_set] -> MATLAB Function2/6(s_dot_set)
  [dl_set] -> MATLAB Function2/7(dl_set)
  MATLAB Function2/1(s_dot2_set) -> [s_dot2_set]
  MATLAB Function2/2(l_dot2_set) -> [l_dot2_set]
  MATLAB Function2/3(ddl_set) -> [ddl_set]
  [s_set] -> Bus Creator/1  "s_set"
  [l_set] -> Bus Creator/2  "l_set"
  [s_dot_set] -> Bus Creator/3  "s_dot_set"
  [l_dot_set] -> Bus Creator/4  "l_dot_set"
  [dl_set] -> Bus Creator/5  "dl_set"
  [s_dot2_set] -> Bus Creator/6  "s_dot2_set"
  [l_dot2_set] -> Bus Creator/7  "l_dot2_set"
  [ddl_set] -> Bus Creator/8  "ddl_set"
  Bus Creator/1 -> Cartesian2FrenetOut/1

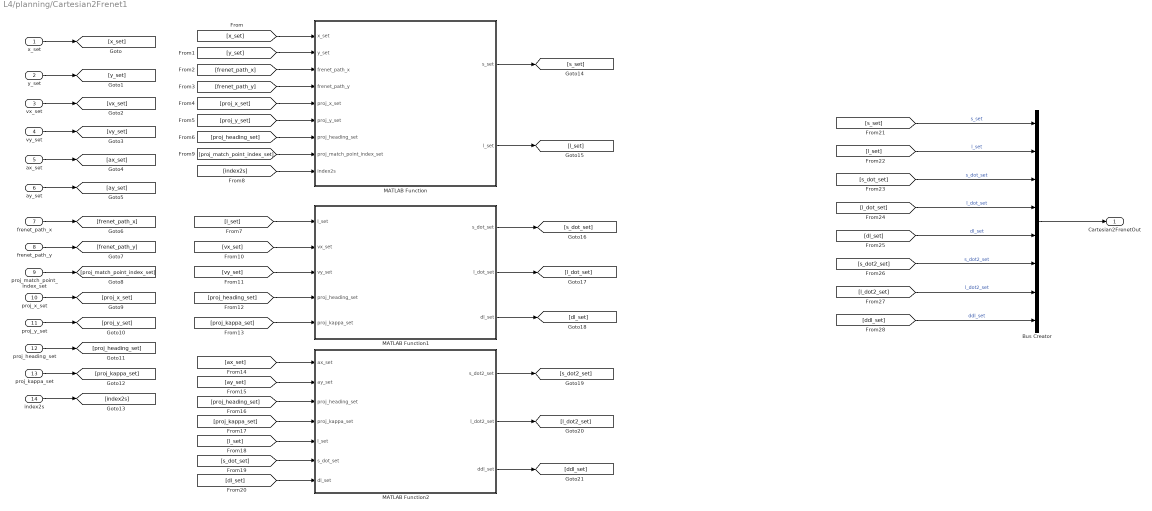
== system L4/planning/Cartesian2Frenet1 ==
  x_set : Inport
  y_set : Inport  Port=2
  vx_set : Inport  Port=3
  vy_set : Inport  Port=4
  ax_set : Inport  Port=5
  ay_set : Inport  Port=6
  frenet_path_x : Inport  Port=7
  frenet_path_y : Inport  Port=8
  proj_match_point_index_set : Inport  Port=9
  proj_x_set : Inport  Port=10
  proj_y_set : Inport  Port=11
  proj_heading_set : Inport  Port=12
  proj_kappa_set : Inport  Port=13
  index2s : Inport  Port=14
  Bus Creator : BusCreator  Inputs=8
  MATLAB Function : MATLAB Function  TreatAsAtomicUnit=on
  MATLAB Function1 : MATLAB Function  TreatAsAtomicUnit=on
  MATLAB Function2 : MATLAB Function  TreatAsAtomicUnit=on
  Cartesian2FrenetOut : Outport
  wires:
  Bus Creator/1 -> Cartesian2FrenetOut/1
  [ddl_set] -> Bus Creator/8  "ddl_set"
  [l_dot2_set] -> Bus Creator/7  "l_dot2_set"
  [s_dot2_set] -> Bus Creator/6  "s_dot2_set"
  [dl_set] -> Bus Creator/5  "dl_set"
  [l_dot_set] -> Bus Creator/4  "l_dot_set"
  [s_dot_set] -> Bus Creator/3  "s_dot_set"
  [l_set] -> Bus Creator/2  "l_set"
  [s_set] -> Bus Creator/1  "s_set"
  MATLAB Function2/3(ddl_set) -> [ddl_set]
  MATLAB Function2/2(l_dot2_set) -> [l_dot2_set]
  MATLAB Function2/1(s_dot2_set) -> [s_dot2_set]
  [dl_set] -> MATLAB Function2/7(dl_set)
  [s_dot_set] -> MATLAB Function2/6(s_dot_set)
  MATLAB Function1/3(dl_set) -> [dl_set]
  MATLAB Function1/2(l_dot_set) -> [l_dot_set]
  MATLAB Function1/1(s_dot_set) -> [s_dot_set]
  [l_set] -> MATLAB Function2/5(l_set)
  [proj_kappa_set] -> MATLAB Function2/4(proj_kappa_set)
  [proj_heading_set] -> MATLAB Function2/3(proj_heading_set)
  [ay_set] -> MATLAB Function2/2(ay_set)
  [ax_set] -> MATLAB Function2/1(ax_set)
  [proj_kappa_set] -> MATLAB Function1/5(proj_kappa_set)
  [proj_heading_set] -> MATLAB Function1/4(proj_heading_set)
  [vy_set] -> MATLAB Function1/3(vy_set)
  [vx_set] -> MATLAB Function1/2(vx_set)
  [l_set] -> MATLAB Function1/1(l_set)
  MATLAB Function/2(l_set) -> [l_set]
  MATLAB Function/1(s_set) -> [s_set]
  [index2s] -> MATLAB Function/9(index2s)
  [proj_heading_set] -> MATLAB Function/7(proj_heading_set)
  [proj_y_set] -> MATLAB Function/6(proj_y_set)
  [proj_match_point_index_set] -> MATLAB Function/8(proj_match_point_index_set)
  [proj_x_set] -> MATLAB Function/5(proj_x_set)
  [frenet_path_y] -> MATLAB Function/4(frenet_path_y)
  [frenet_path_x] -> MATLAB Function/3(frenet_path_x)
  [y_set] -> MATLAB Function/2(y_set)
  [x_set] -> MATLAB Function/1(x_set)
  index2s/1 -> [index2s]
  proj_kappa_set/1 -> [proj_kappa_set]
  proj_heading_set/1 -> [proj_heading_set]
  proj_y_set/1 -> [proj_y_set]
  proj_x_set/1 -> [proj_x_set]
  proj_match_point_index_set/1 -> [proj_match_point_index_set]
  frenet_path_y/1 -> [frenet_path_y]
  frenet_path_x/1 -> [frenet_path_x]
  ay_set/1 -> [ay_set]
  ax_set/1 -> [ax_set]
  vy_set/1 -> [vy_set]
  vx_set/1 -> [vx_set]
  y_set/1 -> [y_set]
  x_set/1 -> [x_set]

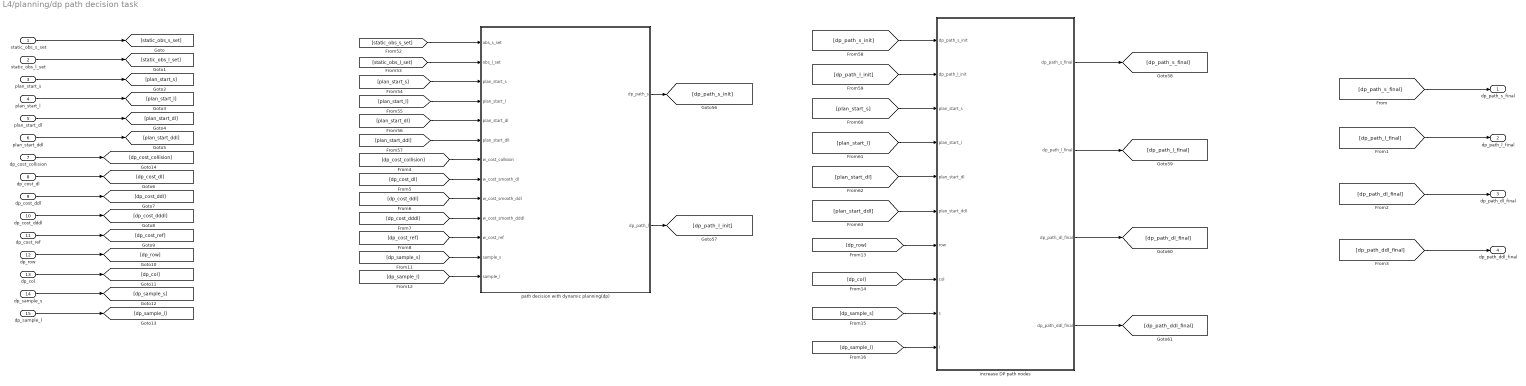
== system L4/planning/dp path decision task ==
  static_obs_s_set : Inport
  static_obs_l_set : Inport  Port=2
  plan_start_s : Inport  Port=3
  plan_start_l : Inport  Port=4
  plan_start_dl : Inport  Port=5
  plan_start_ddl : Inport  Port=6
  dp_cost_collision : Inport  Port=7
  dp_cost_dl : Inport  Port=8
  dp_cost_ddl : Inport  Port=9
  dp_cost_dddl : Inport  Port=10
  dp_cost_ref : Inport  Port=11
  dp_row : Inport  Port=12
  dp_col : Inport  Port=13
  dp_sample_s : Inport  Port=14
  dp_sample_l : Inport  Port=15
  increase DP path nodes : MATLAB Function  TreatAsAtomicUnit=on
  path decision with dynamic planning(dp) : MATLAB Function  TreatAsAtomicUnit=on
  dp_path_s_final : Outport
  dp_path_l_final : Outport  Port=2
  dp_path_dl_final : Outport  Port=3
  dp_path_ddl_final : Outport  Port=4
  wires:
  [plan_start_s] -> path decision with dynamic planning(dp)/3(plan_start_s)
  path decision with dynamic planning(dp)/1(dp_path_s) -> [dp_path_s_init]
  increase DP path nodes/2(dp_path_l_final) -> [dp_path_l_final]
  [static_obs_l_set] -> path decision with dynamic planning(dp)/2(obs_l_set)
  [plan_start_ddl] -> path decision with dynamic planning(dp)/6(plan_start_dll)
  [plan_start_l] -> path decision with dynamic planning(dp)/4(plan_start_l)
  [static_obs_s_set] -> path decision with dynamic planning(dp)/1(obs_s_set)
  [plan_start_dl] -> increase DP path nodes/5(plan_start_dl)
  increase DP path nodes/4(dp_path_ddl_final) -> [dp_path_ddl_final]
  increase DP path nodes/1(dp_path_s_final) -> [dp_path_s_final]
  increase DP path nodes/3(dp_path_dl_final) -> [dp_path_dl_final]
  path decision with dynamic planning(dp)/2(dp_path_l) -> [dp_path_l_init]
  [plan_start_l] -> increase DP path nodes/4(plan_start_l)
  [plan_start_ddl] -> increase DP path nodes/6(plan_start_ddl)
  [plan_start_dl] -> path decision with dynamic planning(dp)/5(plan_start_dl)
  [plan_start_s] -> increase DP path nodes/3(plan_start_s)
  [dp_path_l_init] -> increase DP path nodes/2(dp_path_l_init)
  [dp_path_s_init] -> increase DP path nodes/1(dp_path_s_init)
  static_obs_s_set/1 -> [static_obs_s_set]
  static_obs_l_set/1 -> [static_obs_l_set]
  plan_start_s/1 -> [plan_start_s]
  plan_start_l/1 -> [plan_start_l]
  plan_start_dl/1 -> [plan_start_dl]
  plan_start_ddl/1 -> [plan_start_ddl]
  [dp_path_s_final] -> dp_path_s_final/1
  [dp_path_l_final] -> dp_path_l_final/1
  [dp_path_dl_final] -> dp_path_dl_final/1
  [dp_path_ddl_final] -> dp_path_ddl_final/1
  [dp_cost_collision] -> path decision with dynamic planning(dp)/7(w_cost_collision)
  [dp_cost_dl] -> path decision with dynamic planning(dp)/8(w_cost_smooth_dl)
  [dp_cost_ddl] -> path decision with dynamic planning(dp)/9(w_cost_smooth_ddl)
  [dp_cost_dddl] -> path decision with dynamic planning(dp)/10(w_cost_smooth_dddl)
  [dp_cost_ref] -> path decision with dynamic planning(dp)/11(w_cost_ref)
  [dp_sample_s] -> path decision with dynamic planning(dp)/12(sample_s)
  [dp_sample_l] -> path decision with dynamic planning(dp)/13(sample_l)
  dp_cost_dl/1 -> [dp_cost_dl]
  dp_cost_ddl/1 -> [dp_cost_ddl]
  dp_cost_dddl/1 -> [dp_cost_dddl]
  dp_cost_ref/1 -> [dp_cost_ref]
  dp_row/1 -> [dp_row]
  dp_col/1 -> [dp_col]
  dp_sample_l/1 -> [dp_sample_l]
  dp_sample_s/1 -> [dp_sample_s]
  dp_cost_collision/1 -> [dp_cost_collision]
  [dp_row] -> increase DP path nodes/7(row)
  [dp_col] -> increase DP path nodes/8(col)
  [dp_sample_s] -> increase DP path nodes/9(s)
  [dp_sample_l] -> increase DP path nodes/10(l)
